simulink model "penduldublu_pin"  (R2022b)
settings: Solver=VariableStepAuto  StartTime=0.0  StopTime=10.0  RelTol=1e-3
settings Model: Creator=samue  LastModifiedBy=samue

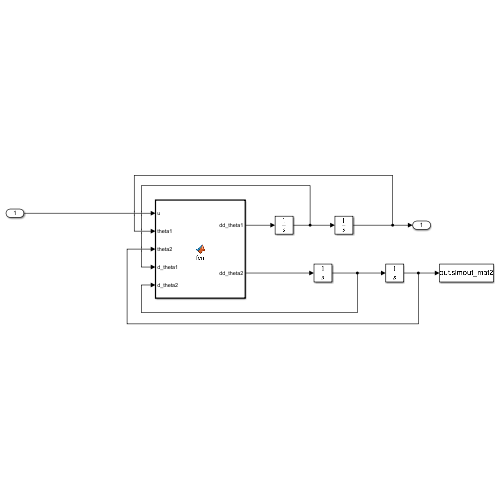
[thumbnail: Simulink's stored preview of the top-level diagram]
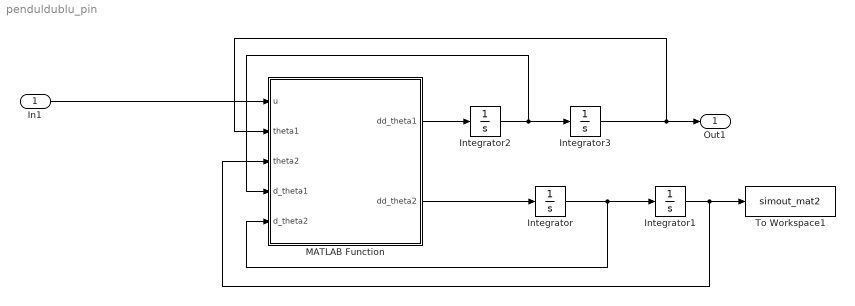
== system penduldublu_pin ==
  In1 : Inport
  Integrator{,1..3} (4 alike) : Integrator
  MATLAB Function : MATLAB Function  TreatAsAtomicUnit=on
  To Workspace1 : ToWorkspace  VariableName=simout_mat2  SampleTime=-1
      settings: Save2DSignal=2-D array (concatenate along first dimension)
  Out1 : Outport
  wires:
  MATLAB Function/1(dd_theta1) -> Integrator2/1
  Integrator/1 -> Integrator1/1, MATLAB Function/5(d_theta2)
  In1/1 -> MATLAB Function/1(u)
  Integrator3/1 -> Out1/1, MATLAB Function/2(theta1)
  Integrator2/1 -> MATLAB Function/4(d_theta1), Integrator3/1
  MATLAB Function/2(dd_theta2) -> Integrator/1
  Integrator1/1 -> To Workspace1/1, MATLAB Function/3(theta2)

== matlab function penduldublu_pin/MATLAB Function ==
  data: u input; dd_theta1 output; theta1 input; theta2 input; d_theta1 input; d_theta2 input; dd_theta2 output
function [dd_theta1,dd_theta2] = fcn(u, theta1,theta2,d_theta1,d_theta2)
zeta = 0.7;
g = 10;
m = 5;
l = 1;

A = - (d_theta2^2) * sin(theta1 - theta2)   - 2 *g*sin(theta1)/l - zeta*d_theta1 + u/(m*l*l);
B =  (d_theta1^2 ) * sin(theta1 - theta2) - g*sin(theta2)/l - zeta*d_theta2;

dd_theta1 = (B* cos( theta1 - theta2)  - A )/( - cos(2*(theta1 - theta2)));
dd_theta2 = (2*B -A* cos( theta1 - theta2)    )/( cos(2*(theta1 - theta2)) );
